simulink library "socmemlib"  (R2021a)
settings: Solver=VariableStepAuto  StartTime=0.0  StopTime=10.0  RelTol=1e-3
PreLoadFcn:
  | soc.internal.HWSWMessageTypeDef();
  | hsb.blkcb2.defineTypes;
undefined symbols (not defined in the file or in its folder): BurstRequest2BusObj, gcbh, hsb, m, ReadAccessBusObj, rearb, RegA, sendFifoFreeMsg, soc, WriteAccessBusObj
libraries: socmemlib_internal x59, priv_hsblib_beta2 x34, socsharedlib_internal x2, socqueuelib_internal x1, simulink x1
(part 5 of 5)

== stateflow chart socmemlib/Memory Channel/Reader 1/From Memory Channel/Streaming Video From Memory Channel/Channel Streaming Master Interface/A4S Master BFM ==
  settings: updateMethod=DISCRETE  sampleTime=ChFrameSampleTime  enableNonTerminalStates=1
  note: NOTE: Trying to use junctions instead
      | of state for 'nextGather' resulted in some
      | funky back-tracing where both transitions of
      | junction outputs were executed.
  note: NOTE: Should we make read requests either when gather buffer processed OR on a time tick?
      | If only on needed event, can combine the sendrdreq and gather sub-charts.
  state fullchart
    state workChart2 [parallel]
      settings: executionOrder=2
      state init
        entry:
        packDataOut = zeros(ChFrameGatherBufferSize, 1, 'uint8');
        ctrl.valid = false;
        ctrl.hEnd = false;
        ctrl.vEnd = false;
        currLineCount = 0;
        currPixelCount = 0;
      note: Ugh!
          | Works, but lose dimensions:
          | zeros(ChLength, ChCompLength, 'like', exemplarChDatum);
          | NOT WORKING (thinks has var dims!!)
          | zeros(ChDimensions, 'like', exemplarChDatum);
      state newFrame
        entry:
        gatherBuffer = zeros(ChGatherBufferSize, 1, 'uint8');
      state drivenotvalid
        entry:
        ctrl.valid = false;
        ctrl.hEnd = false;
        ctrl.vEnd = false;
      state gather
        entry:
        gatherBuffer(gatherBufferIndex:gatherBufferIndex+BurstSize-1) = rdResult.data.rdata(1:rdResult.data.size);
        gatherBufferIndex = gatherBufferIndex + BurstSize;
        gatheredCount = gatheredCount+1;
        RdReqInFlight = RdReqInFlight - 1;
      state driveValidData
        entry:
        gatheredCount = gatheredCount+1;
        %pixel(1:end) = convertData(gatherBuffer(gatherBufferIndex:gatherBufferIndex+ChFrameGatherBufferSize-1), ...
        %   exemplarChContainerDatum, exemplarChDatum);
        packDataOut(1:end) = gatherBuffer(gatherBufferIndex:gatherBufferIndex+ChFrameGatherBufferSize-1);
        gatherBufferIndex = gatherBufferIndex + ChFrameGatherBufferSize;
        currPixelCount = currPixelCount+ChLength;
        ctrl.valid = true;
        ctrl.hStart = false; ctrl.hEnd = false; ctrl.vStart = false; ctrl.vEnd = false;
        inactiveClockCount = 0;
        if (currPixelCount <= ChLength)
        ctrl.hStart = true; ctrl.vStart = true;
        end
        if (rem(currPixelCount-ChLength, ActivePixelsPerLine) == 0)
        ctrl.hStart = true;
        end
        if (rem(currPixelCount, ActivePixelsPerLine) == 0) % REQUIRES LINE ALIGNMENT FOR DIMENSIONS
        ctrl.hEnd = true;
        inactiveClockCount = PorchCount;
        end
        if (currPixelCount >= ChTLASTCount) % REQUIRES FRAME ALIGNMENT FOR DIMENSIONS
        ctrl.hEnd = true; ctrl.vEnd = true;
        currPixelCount = 0;
        inactiveClockCount = PorchCount + BlankingCount*(PorchCount+ActivePixelsPerLine);
        end
      state nextGather
      state aboutToWait
      state waitForNClocks
        entry:
        ctrl.valid = false;
        ctrl.hStart = false; ctrl.hEnd = false;
        ctrl.vStart = false; ctrl.vEnd = false;
        inactiveClockCount = inactiveClockCount - 1;
      state waitForClock
      state waitForReady
        entry:
        ctrl.valid = false;
      state repeatOrGather
      (default) -> fullchart.workChart2.init
      fullchart.workChart2.init -> newFrame
      nextGather -> newFrame : after(ChFrameSampleTime,sec)
      newFrame -> gather [order 1] : rdResult
      newFrame -> drivenotvalid [order 2]
      drivenotvalid -> gather : rdResult
      gather -> drivenotvalid [order 3]
      gather -> gather [order 2] : rdResult
      gather -> (junction 71) [order 1] : [gatheredCount == ChGatherBufferBurstCount] { gatherBufferIndex = 1; gatheredCount = 0; }
      repeatOrGather -> nextGather [order 1] : [gatheredCount == ChGatherCount]
          | { gatherBufferIndex = 1; gatheredCount = 0; }
      (junction 71) -> driveValidData [order 1] : [ready == true]
      (junction 71) -> waitForReady [order 2]
      waitForReady -> driveValidData : [ready == true]
      waitForClock -> driveValidData : after(ChFrameSampleTime,sec)
      driveValidData -> (junction 133)
      (junction 133) -> aboutToWait [order 1] : [inactiveClockCount > 0 && ChLength == 1 && InsertInactivePixelClocks]
      (junction 133) -> repeatOrGather [order 2]
      waitForNClocks -> aboutToWait [order 1] : [inactiveClockCount > 0]
      aboutToWait -> waitForNClocks : after(ChFrameSampleTime,sec)
      waitForNClocks -> repeatOrGather [order 2]
      repeatOrGather -> waitForClock [order 2] : [ready == true]
      repeatOrGather -> waitForReady [order 3]
    state workChart1 [parallel]
      settings: executionOrder=1
      state init
        entry:
        RdReqInFlight = 0;
      state waitForReqFIFO
      state sendRdRequests
        entry:
        burstNum = burstNum+1;
        reqAddr = -1;
        %First burst of every frame must untimed
        if  (ChGatherBufferBurstCount > 1) && (mod(burstNum,ChGatherBufferBurstCount) == 1)
        reqAddr = NO_INFLOW_DELAY;
        end
        readFromMem.data = struct('accessID', burstNum, 'addr', reqAddr, 'size', BurstSize);
        send(readFromMem);
        RdReqInFlight = RdReqInFlight + 1;
      (default) -> fullchart.workChart1.init
      fullchart.workChart1.init -> waitForReqFIFO
      waitForReqFIFO -> sendRdRequests : [RdReqInFlight < FIFOAFullDepth]
      sendRdRequests -> waitForReqFIFO [order 1] : [RdReqInFlight >= FIFOAFullDepth]
      sendRdRequests -> sendRdRequests [order 2]
  (default) -> fullchart
  data: ready input; readFromMem output Bus: ReadAccessBusObj; packDataOut output uint8 size=ChFrameGatherBufferSize; ctrl output Bus: pixelcontrol; rdResult input Bus: ReadAccessBusObj; BurstSize parameter; ChFrameSampleTime parameter; ChGatherBufferBurstCount parameter; ChGatherBufferSize parameter; ChGatherCount parameter; ChLength parameter; burstNum local =0; gatherBuffer local; gatherBufferIndex local =1; gatheredCount local =0; RdReqInFlight local; currPixelCount local =1; currLineCount local; inactiveClockCount local; InsertInactivePixelClocks parameter; ActivePixelsPerLine parameter; BlankingCount parameter; ChFrameGatherBufferSize parameter; ChTLASTCount parameter; PorchCount parameter; FIFOAFullDepth parameter; reqAddr local; NO_INFLOW_DELAY constant double =-2

== stateflow chart socmemlib/Memory Channel/Reader 1/From Memory Channel/Streaming Video From Memory Channel with Fsync/Channel Streaming Master Interface/A4S Master BFM ==
  settings: updateMethod=DISCRETE  sampleTime=ChFrameSampleTime  enableNonTerminalStates=1
  note: NOTE: Trying to use junctions instead
      | of state for 'nextGather' resulted in some
      | funky back-tracing where both transitions of
      | junction outputs were executed.
  note: NOTE: Should we make read requests either when gather buffer processed OR on a time tick?
      | If only on needed event, can combine the sendrdreq and gather sub-charts.
  state fullchart
    state workChart2 [parallel]
      settings: executionOrder=2
      state init
        entry:
        packDataOut = zeros(ChFrameGatherBufferSize, 1, 'uint8');
        ctrl.valid = false;
        ctrl.hEnd = false;
        ctrl.vEnd = false;
        currLineCount = 0;
        currPixelCount = 0;
      note: Ugh!
          | Works, but lose dimensions:
          | zeros(ChLength, ChCompLength, 'like', exemplarChDatum);
          | NOT WORKING (thinks has var dims!!)
          | zeros(ChDimensions, 'like', exemplarChDatum);
      state newFrame
        entry:
        gatherBuffer = zeros(ChGatherBufferSize, 1, 'uint8');
      state drivenotvalid
        entry:
        ctrl.valid = false;
        ctrl.hEnd = false;
        ctrl.vEnd = false;
      state gather
        entry:
        gatherBuffer(gatherBufferIndex:gatherBufferIndex+BurstSize-1) = rdResult.data.rdata(1:rdResult.data.size);
        gatherBufferIndex = gatherBufferIndex + BurstSize;
        gatheredCount = gatheredCount+1;
        RdReqInFlight = RdReqInFlight - 1;
      state driveValidData
        entry:
        gatheredCount = gatheredCount+1;
        %pixel(1:end) = convertData(gatherBuffer(gatherBufferIndex:gatherBufferIndex+ChFrameGatherBufferSize-1), ...
        %   exemplarChContainerDatum, exemplarChDatum);
        packDataOut(1:end) = gatherBuffer(gatherBufferIndex:gatherBufferIndex+ChFrameGatherBufferSize-1);
        gatherBufferIndex = gatherBufferIndex + ChFrameGatherBufferSize;
        currPixelCount = currPixelCount+ChLength;
        ctrl.valid = true;
        ctrl.hStart = false; ctrl.hEnd = false; ctrl.vStart = false; ctrl.vEnd = false;
        inactiveClockCount = 0;
        if (currPixelCount <= ChLength)
        ctrl.hStart = true; ctrl.vStart = true;
        end
        if (rem(currPixelCount-ChLength, ActivePixelsPerLine) == 0)
        ctrl.hStart = true;
        end
        if (rem(currPixelCount, ActivePixelsPerLine) == 0) % REQUIRES LINE ALIGNMENT FOR DIMENSIONS
        ctrl.hEnd = true;
        inactiveClockCount = PorchCount;
        end
        if (currPixelCount >= ChTLASTCount) % REQUIRES FRAME ALIGNMENT FOR DIMENSIONS
        ctrl.hEnd = true; ctrl.vEnd = true;
        currPixelCount = 0;
        inactiveClockCount = PorchCount + BlankingCount*(PorchCount+ActivePixelsPerLine);
        end
      state nextGather
      state aboutToWait
      state waitForNClocks
        entry:
        ctrl.valid = false;
        ctrl.hStart = false; ctrl.hEnd = false;
        ctrl.vStart = false; ctrl.vEnd = false;
        inactiveClockCount = inactiveClockCount - 1;
      state waitForClock
      state waitForReady
        entry:
        ctrl.valid = false;
      state repeatOrGather
      (default) -> fullchart.workChart2.init
      fullchart.workChart2.init -> newFrame
      nextGather -> newFrame : after(ChFrameSampleTime, sec)
      newFrame -> gather [order 1] : rdResult
      newFrame -> drivenotvalid [order 2]
      drivenotvalid -> gather : rdResult
      gather -> drivenotvalid [order 3]
      gather -> gather [order 2] : rdResult
      gather -> (junction 71) [order 1] : [gatheredCount == ChGatherBufferBurstCount] { gatherBufferIndex = 1; gatheredCount = 0; }
      repeatOrGather -> nextGather [order 1] : [gatheredCount == ChGatherCount]
          | { gatherBufferIndex = 1; gatheredCount = 0; }
      (junction 71) -> driveValidData [order 1] : [ready == true]
      (junction 71) -> waitForReady [order 2]
      waitForReady -> driveValidData : [ready == true]
      waitForClock -> driveValidData : after(ChFrameSampleTime,sec)
      driveValidData -> (junction 133)
      (junction 133) -> aboutToWait [order 1] : [inactiveClockCount > 0 && ChLength == 1 && InsertInactivePixelClocks]
      (junction 133) -> repeatOrGather [order 2]
      waitForNClocks -> aboutToWait [order 1] : [inactiveClockCount > 0]
      aboutToWait -> waitForNClocks : after(ChFrameSampleTime,sec)
      waitForNClocks -> repeatOrGather [order 2]
      repeatOrGather -> waitForClock [order 2] : [ready == true]
      repeatOrGather -> waitForReady [order 3]
    state workChart1 [parallel]
      settings: executionOrder=1
      state init
        entry:
        RdReqInFlight = 0;
      state waitForReqFIFO
      state sendRdRequests
        entry:
        burstNum = burstNum+1;
        reqAddr = -1;
        %First burst of every frame must untimed
        if  (ChGatherBufferBurstCount > 1) && (mod(burstNum,ChGatherBufferBurstCount) == 1)
        reqAddr = NO_INFLOW_DELAY;
        end
        readFromMem.data = struct('accessID', burstNum, 'addr', reqAddr, 'size', BurstSize);
        send(readFromMem);
        RdReqInFlight = RdReqInFlight + 1;
      (default) -> fullchart.workChart1.init
      fullchart.workChart1.init -> waitForReqFIFO
      waitForReqFIFO -> sendRdRequests : [RdReqInFlight < FIFOAFullDepth]
      sendRdRequests -> waitForReqFIFO [order 1] : [RdReqInFlight >= FIFOAFullDepth]
      sendRdRequests -> sendRdRequests [order 2]
  (default) -> fullchart
  data: ready input; readFromMem output Bus: ReadAccessBusObj; packDataOut output uint8 size=ChFrameGatherBufferSize; ctrl output Bus: pixelcontrol; rdResult input Bus: ReadAccessBusObj; BurstSize parameter; ChFrameGatherBufferSize parameter; ChFrameSampleTime parameter; ChGatherBufferBurstCount parameter; ChGatherBufferSize parameter; ChGatherCount parameter; ChLength parameter; ChTLASTCount parameter; burstNum local =0; gatherBuffer local; gatherBufferIndex local =1; gatheredCount local =0; RdReqInFlight local =0; currPixelCount local =1; currLineCount local; ActivePixelsPerLine parameter; BlankingCount parameter; PorchCount parameter; inactiveClockCount local; InsertInactivePixelClocks parameter; FIFOAFullDepth parameter; reqAddr local; NO_INFLOW_DELAY constant double =-2

== stateflow chart socmemlib/Memory Channel/Reader 1/bufDoneGate/async/Buffer Release Gate ==
  settings: enableNonTerminalStates=1
  state waitForBufDone
  state waitForFrameDone
    entry:
    forward(bufDoneIn, int_bufDone);
  state dequeue_internal
  state forwardBufDone
    entry:
    forward(int_bufDone, bufDoneOut);
  (default) -> waitForBufDone
  forwardBufDone -> waitForBufDone
  waitForBufDone -> waitForFrameDone : bufDoneIn
  waitForFrameDone -> dequeue_internal : frameDone
  dequeue_internal -> forwardBufDone : int_bufDone
  data: bufDoneIn input Bus: BufferRequest2BusObj; frameDone input; bufDoneOut output Bus: BufferRequest2BusObj; int_bufDone local Bus: BufferRequest2BusObj
